simulink model "10_MCU_PMSM1_Trajectoire_dsPIC33CK_LVMC"  (R2023b)
settings: Solver=FixedStepDiscrete  StartTime=0.0  StopTime=10.0  FixedStep=5e-5  RelTol=1e-3  EnableMultiTasking=on
InitFcn:
  | %% Trajectoire Source
  | 
  | t0 = 0;
  | t1 = t0+0.1;
  | t2 = t1+0.1;
  | t3 = t2+0.5;
  | t4 = t3+0.2;
  | t5 = t4+0.5;
  | t6 = t5+0.2;
  | t7 = t6+0.1;
  | 
  | 
  | 
  | x = [t0 t1 t2 t3 t4 t5 t6 t7];
  | y = [0 0 0.25 0.25 1 1 0 0];
  | 
  | 
  | %% Trajectoire charge
  | t0 = 0;
  | t1 = t0+0.4;
  | t2 = t1+1e-2;
  | t3 = t2+0.1;
  | t4 = t3+1e-2;
  | t5 = 1.1;
  | t6 = t5+1e-2;
  | t7 = t6+0.1
  | t8 = t7+1e-2
  | t9 = 1.7;
  | x2 = [t0 t1 t2 t3 t4 t5 t6 t7 t8 t9];
  | y2 = [0 0 1 1 0 0 1 1 0 0];
undefined symbols (not defined in the file or in its folder): A0, A4, AN0, AN1, B0, B2, Bias1, Bias2, C12, C13, C14, C7, control, D11, D12, D13, D14, D5, D6, D7, diff, DiscIntNeverNeededParam, inverter, Max, MaxPer, model, ms, NumBits1, NumBits2, P20, P32, P55, P60, P61, P62, P69, P70, P71, P75, P76, P77, P78, Pin, pmsm, PosRange1, PosRange2, PWM1max, Resol, s, Slope1, Slope2, us
libraries: simulink x55, MCHP_Blockset x26
(part 4 of 4)

== system 10_MCU_PMSM1_Trajectoire_dsPIC33CK_LVMC/Park/Clarke ==
  note: Clark transform
      | $x_{\alpha\beta} = \frac{2}{3}\underbrace{\left[\begin{array}{ccc}1&-\frac{1}{2}&-\frac{1}{2}\\0&\frac{\sqrt{3}}{2}&-\frac{\sqrt{3}}{2}\end{array}\right]}_{C_{23}}x_{abc}$
      | if only 2 currents are measured since $x_a+x_b+x_c = 0$
      | $x_{abc} = \left[\begin{array}{cc}1 & 0\\0 & 1\\-1&-1\end{array}\right]x_{ab}$
      | leading to
      | $x_{\alpha\beta} = \underbrace{\left[\begin{array}{cc}1&0\\\frac{1}{\sqrt{3}}&\frac{2}{\sqrt{3}}\end{array}\right]}_{C_{22}}x_{ab}$
  xab(c) : Inport
  C1 : Gain  Gain=[1/sqrt(3) 2/sqrt(3)]  Multiplication=Matrix(K*u)  OutDataTypeStr=Inherit: Same as input
  Mux : Mux  Inputs=2
  Selector : Selector  InputPortWidth=2  IndexOptions=Index vector (dialog)  Indices=[1]  OutputSizes=1
  xalphabeta : Outport  VectorParamsAs1DForOutWhenUnconnected=off
  wires:
  C1/1 -> Mux/2
  Selector/1 -> Mux/1
  Mux/1 -> xalphabeta/1
  xab(c)/1 -> C1/1, Selector/1

== system 10_MCU_PMSM1_Trajectoire_dsPIC33CK_LVMC/Park/Park ==
  note: Park
      | $x_{dq} = P(\theta)^{-1}x_{\alpha\beta}\\ P(p\theta)^{-1} = \left[\begin{array}{cc}\cos(p\theta) & \sin(p\theta)\\ -\sin(p\theta) & \cos(p\theta) \end{array}\right]$
  xalphabeta : Inport  PortDimensions=2
  P(pth) : Inport  Port=2
  Data Type Duplicate2 : DataTypeDuplicate
  Park : Product  Multiplication=Matrix(*)  OutDataTypeStr=Inherit: Inherit via back propagation  RndMeth=Round
  xdq : Outport  VectorParamsAs1DForOutWhenUnconnected=off
  wires:
  P(pth)/1 -> Park/1
  xalphabeta/1 -> Park/2, Data Type Duplicate2/2
  Park/1 -> xdq/1, Data Type Duplicate2/1

== system 10_MCU_PMSM1_Trajectoire_dsPIC33CK_LVMC/Park inverse/Clarke Inverse ==
  note: Clarke inverse
  xalphabeta : Inport
  C23' : Gain  Gain=|  Multiplication=Matrix(K*u)  OutDataTypeStr=Inherit: Inherit via back propagation  RndMeth=Round
      | [1   -1/2        -1/2;
      |         0   sqrt(3)/2   -sqrt(3)/2]'
  xabc : Outport  VectorParamsAs1DForOutWhenUnconnected=off
  wires:
  xalphabeta/1 -> C23'/1
  C23'/1 -> xabc/1

== system 10_MCU_PMSM1_Trajectoire_dsPIC33CK_LVMC/Park inverse/Park inverse ==
  note: Inverse Park
      | $x_{\alpha\beta} = P(p\theta)x_{dq}\\ P(p\theta) = \left[\begin{array}{cc}\cos(p\theta) & -\sin(p\theta)\\ \sin(p\theta) & \cos(p\theta) \end{array}\right]$
  xdq : Inport
  P(pth) : Inport  Port=2
  Data Type Duplicate2 : DataTypeDuplicate
  Transpose : Math  Operator=transpose
  Transpose1 : Math  Operator=transpose
  xalpha sin(pth)1 : Product  Multiplication=Matrix(*)  OutDataTypeStr=Inherit: Inherit via back propagation  RndMeth=Round
  xalpahbeta : Outport  VectorParamsAs1DForOutWhenUnconnected=off
  wires:
  P(pth)/1 -> xalpha sin(pth)1/2
  Transpose1/1 -> xalpahbeta/1
  Transpose/1 -> Data Type Duplicate2/2, xalpha sin(pth)1/1
  xdq/1 -> Transpose/1
  xalpha sin(pth)1/1 -> Data Type Duplicate2/1, Transpose1/1

== system 10_MCU_PMSM1_Trajectoire_dsPIC33CK_LVMC/Selector/Direction Toggle ==
  in : Inport
  Change when button is pressed : simulink/Logic and Bit Operations/Detect Decrease  vinit=0.0  OutDataTypeStr=uint8
  Logical Operator : Logic  Operator=XOR  AllPortsSameDT=off  OutDataTypeStr=boolean
  Unit Delay : UnitDelay  SampleTime=-1  HasFrameUpgradeWarning=on
  Toggle : Outport  VectorParamsAs1DForOutWhenUnconnected=off
  wires:
  Logical Operator/1 -> Unit Delay/1, Toggle/1  "Toggle"
  in/1 -> Change when button is pressed/1
  Change when button is pressed/1 -> Logical Operator/1
  Unit Delay/1 -> Logical Operator/2

== system 10_MCU_PMSM1_Trajectoire_dsPIC33CK_LVMC/Selector/Mode Toggle ==
  state : Inport
  Bitwise Operator : simulink/Logic and Bit Operations/Bitwise Operator  logicop=AND  UseBitMask=on  BitMask=1  BitMaskRealWorld=Stored Integer
  Change when button is pressed : simulink/Logic and Bit Operations/Detect Decrease  vinit=0.0  OutDataTypeStr=uint8
  Sum : Sum  OutDataTypeStr=uint16  AccumDataTypeStr=uint16
  Unit Delay : UnitDelay  SampleTime=-1  HasFrameUpgradeWarning=on
  Mode : Outport  PortDimensions=1  VectorParamsAs1DForOutWhenUnconnected=off
  wires:
  Change when button is pressed/1 -> Sum/1
  Bitwise Operator/1 -> Mode/1, Unit Delay/1
  Unit Delay/1 -> Sum/2
  Sum/1 -> Bitwise Operator/1
  state/1 -> Change when button is pressed/1

== system 10_MCU_PMSM1_Trajectoire_dsPIC33CK_LVMC/Selector/On//Off Toggle ==
  in : Inport
  Change when button is pressed : simulink/Logic and Bit Operations/Detect Decrease  vinit=0.0  OutDataTypeStr=uint8
  Logical Operator : Logic  Operator=XOR  AllPortsSameDT=off  OutDataTypeStr=boolean
  Unit Delay : UnitDelay  SampleTime=-1  HasFrameUpgradeWarning=on
  Toggle : Outport  VectorParamsAs1DForOutWhenUnconnected=off
  wires:
  Unit Delay/1 -> Logical Operator/2
  Change when button is pressed/1 -> Logical Operator/1
  in/1 -> Change when button is pressed/1
  Logical Operator/1 -> Unit Delay/1, Toggle/1  "Toggle"

== system 10_MCU_PMSM1_Trajectoire_dsPIC33CK_LVMC/Selector/Subsystem1 ==
  Enable : EnablePort  StatesWhenEnabling=reset
  1-D Lookup Table : Lookup_n-D  NumberOfTableDimensions=1  BreakpointsForDimension1=x  Table=y  ExtrapMethod=Clip  InternalRulePriority=Speed  OutDataTypeStr=fixdt(1,16,14)  RndMeth=Simplest
  Constant : Constant  OutDataTypeStr=int16  SampleTime=0.001
  Discrete-Time Integrator : DiscreteIntegrator  SampleTime=0.001  OutDataTypeStr=fixdt(1,32,20)  SaturateOnIntegerOverflow=on  LimitOutput=on  UpperSaturationLimit=100  LowerSaturationLimit=0  ICPrevOutput=DiscIntNeverNeededParam  ICPrevScaledInput=DiscIntNeverNeededParam
  Gain : Gain  Gain=1.7/10  OutMax=[100]  OutDataTypeStr=fixdt(1,16,7)
  Mode1 : Outport
  wires:
  Discrete-Time Integrator/1 -> Gain/1
  Gain/1 -> 1-D Lookup Table/1
  1-D Lookup Table/1 -> Mode1/1
  Constant/1 -> Discrete-Time Integrator/1

== system 10_MCU_PMSM1_Trajectoire_dsPIC33CK_LVMC/Selector/Subsystem2 ==
  In1 : Inport
  Trigger : TriggerPort  VariantControl=(inherit)  PortDimensions=1
  UART Tx : MCHP_Blockset/BUS UART/UART Tx  UART_REF=1  ORDERING=None  AllOrNothing=off  SampleTime=-1  MCHP_MASTERLINK=MCU_logTrajectoire_dsPIC33CK_LVMC/BOARD dsPIC33CK LVMC/Microchip Master  NSend_Input=off  UART_String=off  NSend_Output=off
      settings: SourceProductName=MPLAB Device Blocks for Simulink
  wires:
  In1/1 -> UART Tx/1

== system 10_MCU_PMSM1_Trajectoire_dsPIC33CK_LVMC/Selector/Subsystem3 ==
  In1 : Inport
  Trigger : TriggerPort  TriggerType=falling  VariantControl=(inherit)  PortDimensions=1
  UART Tx : MCHP_Blockset/BUS UART/UART Tx  UART_REF=1  ORDERING=None  AllOrNothing=off  SampleTime=-1  MCHP_MASTERLINK=MCU_logTrajectoire_dsPIC33CK_LVMC/BOARD dsPIC33CK LVMC/Microchip Master  NSend_Input=off  UART_String=off  NSend_Output=off
      settings: SourceProductName=MPLAB Device Blocks for Simulink
  wires:
  In1/1 -> UART Tx/1

== system 10_MCU_PMSM1_Trajectoire_dsPIC33CK_LVMC/BOARD dsPIC33CK LVMC/Center & sign reversal/Downsample Averaged 2000 samples remove bias ==
  note: DownSample & Average by changing data scaling
  In1 : Inport
  Enable : EnablePort
  Compare To Constant : simulink/Logic and Bit Operations/Compare To Constant  relop===  const=1  OutDataTypeStr=boolean
  Counter Limited : simulink/Sources/Counter Limited  uplimit=DownSample-1  tsamp=-1
  Data Type Duplicate : DataTypeDuplicate
  Data Type Propagation : simulink/Signal Attributes/Data Type Propagation  PropDataType=fixdt(1, 16)  IfRefDouble=double  IfRefSingle=single  IsSigned=IsSigned1 or IsSigned2  NumBitsBase=NumBits1+NumBits2  NumBitsMult=1  NumBitsAdd=0  NumBitsAllowFinal=1:128  PropScaling=2^-10  ValuesUsedBestPrec=[5 -7]  SlopeBase=Slope1  SlopeMult=1  SlopeAdd=0  BiasBase=Bias1  BiasMult=1  BiasAdd=0
  Data Type Propagation1 : simulink/Signal Attributes/Data Type Propagation  PropDataType=fixdt(1, 16)  IfRefDouble=double  IfRefSingle=single  IsSigned=IsSigned1 or IsSigned2  NumBitsBase=NumBits1+NumBits2  NumBitsMult=1  NumBitsAdd=0  NumBitsAllowFinal=1:128  PropScaling=2^-10  ValuesUsedBestPrec=[5 -7]  SlopeBase=PosRange1  SlopeMult=1  SlopeAdd=0  BiasBase=Bias1  BiasMult=1  BiasAdd=0
  Discrete-Time Integrator : DiscreteIntegrator  IntegratorMethod=Accumulation: Backward Euler  gainval=1  ExternalReset=sampled level  SampleTime=-1  OutDataTypeStr=Inherit: Inherit via back propagation  ICPrevOutput=DiscIntNeverNeededParam  ICPrevScaledInput=DiscIntNeverNeededParam
  Gain : Gain  Gain=1/DownSample  OutDataTypeStr=Inherit: Inherit via back propagation  RndMeth=Round
  Gain1 : Gain  Gain=1/DownSample  OutDataTypeStr=Inherit: Inherit via back propagation
  Rate Transition1 : RateTransition  OutPortSampleTimeOpt=Multiple of input port sample time  OutPortSampleTimeMultiple=DownSample  OutPortSampleTime=DownSample
  Rate Transition3 : RateTransition  OutPortSampleTimeOpt=Multiple of input port sample time  OutPortSampleTimeMultiple=DownSample  OutPortSampleTime=DownSample
  Terminator : Terminator
  Out1 : Outport  VectorParamsAs1DForOutWhenUnconnected=off
  wires:
  Gain1/1 -> Data Type Propagation1/3, Terminator/1
  Rate Transition1/1 -> Data Type Duplicate/1, Data Type Propagation1/1, Data Type Propagation1/2
  Gain/1 -> Out1/1, Data Type Duplicate/2
  Counter Limited/1 -> Compare To Constant/1
  Discrete-Time Integrator/1 -> Rate Transition3/1, Data Type Propagation/3
  Compare To Constant/1 -> Discrete-Time Integrator/2
  In1/1 -> Data Type Propagation/1, Data Type Propagation/2, Discrete-Time Integrator/1, Rate Transition1/1
  Rate Transition3/1 -> Gain/1, Gain1/1

== system 10_MCU_PMSM1_Trajectoire_dsPIC33CK_LVMC/BOARD dsPIC33CK LVMC/Timing Analysis/Downsample Averaged2 ==
  note: DownSample & Average by changing data scaling
  In1 : Inport
  Compare To Constant : simulink/Logic and Bit Operations/Compare To Constant  relop===  const=1  OutDataTypeStr=boolean
  Counter Limited : simulink/Sources/Counter Limited  uplimit=DownSample-1  tsamp=-1
  Data Type Duplicate : DataTypeDuplicate
  Data Type Propagation : simulink/Signal Attributes/Data Type Propagation  PropDataType=fixdt(1, 16)  IfRefDouble=double  IfRefSingle=single  IsSigned=IsSigned1 or IsSigned2  NumBitsBase=NumBits1+NumBits2  NumBitsMult=1  NumBitsAdd=0  NumBitsAllowFinal=1:128  PropScaling=2^-10  ValuesUsedBestPrec=[5 -7]  SlopeBase=Slope1  SlopeMult=1  SlopeAdd=0  BiasBase=Bias1  BiasMult=1  BiasAdd=0
  Data Type Propagation1 : simulink/Signal Attributes/Data Type Propagation  PropDataType=fixdt(1, 16)  IfRefDouble=double  IfRefSingle=single  IsSigned=IsSigned1 or IsSigned2  NumBitsBase=NumBits1+NumBits2  NumBitsMult=1  NumBitsAdd=0  NumBitsAllowFinal=1:128  PropScaling=2^-10  ValuesUsedBestPrec=[5 -7]  SlopeBase=PosRange1  SlopeMult=1  SlopeAdd=0  BiasBase=Bias1  BiasMult=1  BiasAdd=0
  Discrete-Time Integrator : DiscreteIntegrator  IntegratorMethod=Accumulation: Backward Euler  gainval=1  ExternalReset=sampled level  SampleTime=-1  OutDataTypeStr=Inherit: Inherit via back propagation  ICPrevOutput=DiscIntNeverNeededParam  ICPrevScaledInput=DiscIntNeverNeededParam
  Gain : Gain  Gain=1/DownSample  OutDataTypeStr=Inherit: Inherit via back propagation
  Gain1 : Gain  Gain=1/DownSample  OutDataTypeStr=Inherit: Inherit via back propagation
  Rate Transition1 : RateTransition  Deterministic=off  OutPortSampleTime=[InputSampleTime * DownSample]
  Rate Transition3 : RateTransition  OutPortSampleTime=[InputSampleTime * DownSample]
  Terminator : Terminator
  Out1 : Outport  VectorParamsAs1DForOutWhenUnconnected=off
  wires:
  Rate Transition3/1 -> Gain1/1, Gain/1
  In1/1 -> Discrete-Time Integrator/1, Rate Transition1/1, Data Type Propagation/2, Data Type Propagation/1
  Compare To Constant/1 -> Discrete-Time Integrator/2
  Discrete-Time Integrator/1 -> Data Type Propagation/3, Rate Transition3/1
  Counter Limited/1 -> Compare To Constant/1
  Gain/1 -> Data Type Duplicate/2, Out1/1
  Rate Transition1/1 -> Data Type Propagation1/2, Data Type Propagation1/1, Data Type Duplicate/1
  Gain1/1 -> Data Type Propagation1/3, Terminator/1

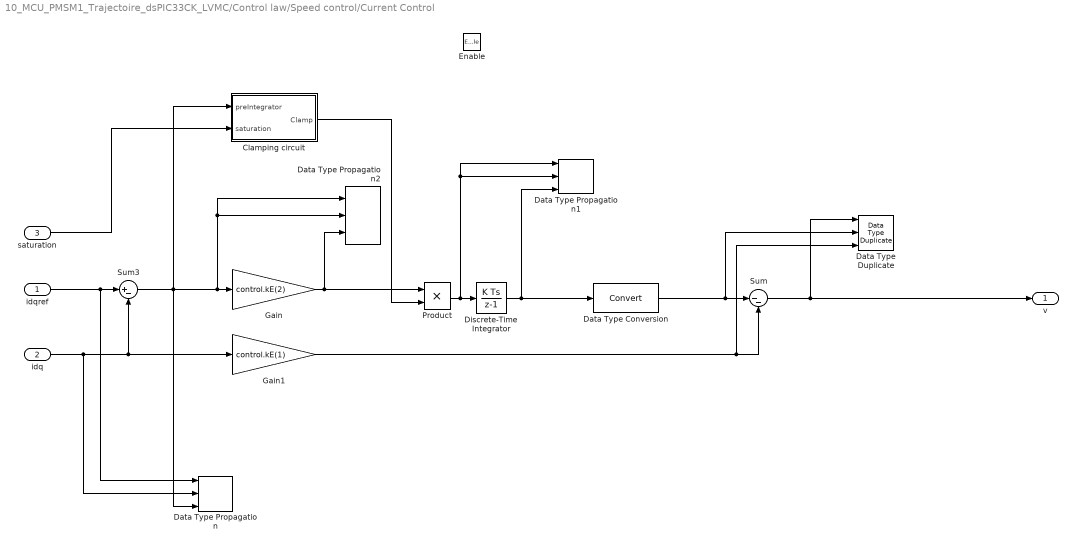
== system 10_MCU_PMSM1_Trajectoire_dsPIC33CK_LVMC/Control law/Speed control/Current Control ==
  idqref : Inport
  idq : Inport  Port=2
  saturation : Inport  Port=3
  Enable : EnablePort  StatesWhenEnabling=reset
  Clamping circuit : Subsystem
  Data Type Duplicate : DataTypeDuplicate  NumInputPorts=3
  Data Type Propagation : simulink/Signal Attributes/Data Type Propagation  PropDataType=fixdt(1, 16)  IfRefDouble=double  IfRefSingle=single  IsSigned=IsSigned1 or IsSigned2  NumBitsBase=max([NumBits1 NumBits2])  NumBitsMult=1  NumBitsAdd=0  NumBitsAllowFinal=1:128  PropScaling=2^-(15-ceil(log2(2*inverter.iMax)))  ValuesUsedBestPrec=[5 -7]  SlopeBase=max([PosRange1 PosRange2])  SlopeMult=2  SlopeAdd=0  BiasBase=Bias1  BiasMult=1  BiasAdd=0
  Data Type Propagation1 : simulink/Signal Attributes/Data Type Propagation  PropDataType=fixdt(1, 16)  IfRefDouble=single  IfRefSingle=single  IsSigned=IsSigned1 or IsSigned2  NumBitsBase=NumBits1+NumBits2  NumBitsMult=1  NumBitsAdd=0  NumBitsAllowFinal=1:128  PropScalingMode=Specify via dialog  PropScaling=2^-23  ValuesUsedBestPrec=[5 -7]  SlopeBase=min([Slope1 Slope2])  SlopeMult=1  SlopeAdd=0  BiasBase=Bias1  BiasMult=1  BiasAdd=0
  Data Type Propagation2 : simulink/Signal Attributes/Data Type Propagation  PropDataType=fixdt(1, 16)  IfRefDouble=double  IfRefSingle=single  IsSigned=TRUE  NumBitsBase=max([NumBits1 NumBits2])  NumBitsMult=1  NumBitsAdd=0  NumBitsAllowFinal=[1:128]  PropScaling=2^-(15-ceil(log2(inverter.vDC/sqrt(3))))  ValuesUsedBestPrec=[100 -100]  SlopeBase=max([PosRange1 PosRange2])  SlopeMult=abs(control.kE(2))  SlopeAdd=0  BiasBase=Bias1  BiasMult=1  BiasAdd=0
  Data Type Conversion : DataTypeConversion  SaturateOnIntegerOverflow=off  RndMeth=Floor
  Discrete-Time Integrator : DiscreteIntegrator  SampleTime=-1  OutDataTypeStr=Inherit: Inherit via back propagation  SaturateOnIntegerOverflow=on  ICPrevOutput=DiscIntNeverNeededParam  ICPrevScaledInput=DiscIntNeverNeededParam
  Gain : Gain  Gain=control.kE(2)  OutDataTypeStr=Inherit: Inherit via back propagation  SaturateOnIntegerOverflow=on
  Gain1 : Gain  Gain=control.kE(1)  OutDataTypeStr=Inherit: Inherit via back propagation  SaturateOnIntegerOverflow=on
  Product : Product  OutDataTypeStr=Inherit: Same as first input
  Sum : Sum  Inputs=|--  OutDataTypeStr=Inherit: Inherit via back propagation  SaturateOnIntegerOverflow=on
  Sum3 : Sum  Inputs=|+-  OutDataTypeStr=Inherit: Inherit via back propagation  SaturateOnIntegerOverflow=on
  v : Outport  VectorParamsAs1DForOutWhenUnconnected=off
  wires:
  Data Type Conversion/1 -> Sum/1, Data Type Duplicate/2
  Sum/1 -> v/1, Data Type Duplicate/1
  idqref/1 -> Sum3/1, Data Type Propagation/1
  idq/1 -> Sum3/2, Gain1/1, Data Type Propagation/2
  Discrete-Time Integrator/1 -> Data Type Conversion/1, Data Type Propagation1/3
  Gain1/1 -> Sum/2, Data Type Duplicate/3
  saturation/1 -> Clamping circuit/2(saturation)
  Product/1 -> Data Type Propagation1/2, Data Type Propagation1/1, Discrete-Time Integrator/1
  Clamping circuit/1(Clamp) -> Product/2
  Gain/1 -> Data Type Propagation2/3, Product/1
  Sum3/1 -> Gain/1, Data Type Propagation2/2, Data Type Propagation2/1, Data Type Propagation/3, Clamping circuit/1(preIntegrator)

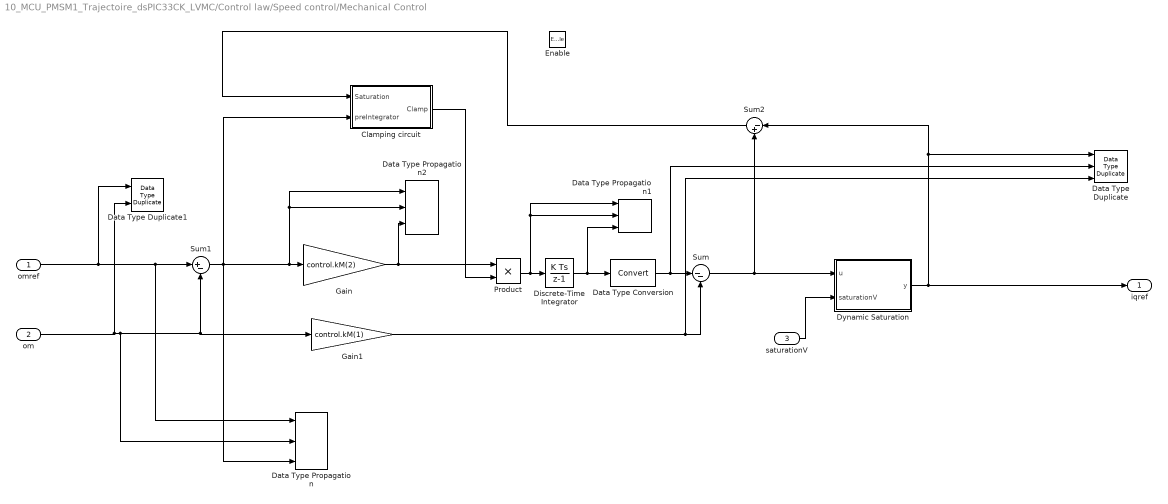
== system 10_MCU_PMSM1_Trajectoire_dsPIC33CK_LVMC/Control law/Speed control/Mechanical Control ==
  omref : Inport
  om : Inport  Port=2
  saturationV : Inport  Port=3
  Enable : EnablePort  StatesWhenEnabling=reset
  Clamping circuit : Subsystem
  Data Type Duplicate : DataTypeDuplicate  NumInputPorts=3
  Data Type Duplicate1 : DataTypeDuplicate
  Data Type Propagation : simulink/Signal Attributes/Data Type Propagation  PropDataType=fixdt(1, 16)  IfRefDouble=double  IfRefSingle=single  IsSigned=IsSigned1 or IsSigned2  NumBitsBase=max([NumBits1 NumBits2])  NumBitsMult=1  NumBitsAdd=0  NumBitsAllowFinal=1:128  PropScaling=2^-(15-ceil(log2(2*pmsm.omegaMax)))  ValuesUsedBestPrec=[5 -7]  SlopeBase=max([PosRange1 PosRange2])  SlopeMult=2  SlopeAdd=0  BiasBase=Bias1  BiasMult=1  BiasAdd=0
  Data Type Propagation1 : simulink/Signal Attributes/Data Type Propagation  PropDataType=fixdt(1, 16)  IfRefDouble=single  IfRefSingle=single  IsSigned=IsSigned1 or IsSigned2  NumBitsBase=NumBits1+NumBits2  NumBitsMult=1  NumBitsAdd=0  NumBitsAllowFinal=1:128  PropScalingMode=Specify via dialog  PropScaling=2^-23  ValuesUsedBestPrec=[5 -7]  SlopeBase=min([Slope1 Slope2])  SlopeMult=1  SlopeAdd=0  BiasBase=Bias1  BiasMult=1  BiasAdd=0
  Data Type Propagation2 : simulink/Signal Attributes/Data Type Propagation  PropDataType=fixdt(1, 16)  IfRefDouble=double  IfRefSingle=single  IsSigned=TRUE  NumBitsBase=max([NumBits1 NumBits2])  NumBitsMult=1  NumBitsAdd=0  NumBitsAllowFinal=[1:128]  PropScaling=2^-(15-ceil(log2(inverter.vDC/sqrt(3))))  ValuesUsedBestPrec=[100 -100]  SlopeBase=max([PosRange1 PosRange2])  SlopeMult=abs(control.kM(2))  SlopeAdd=0  BiasBase=Bias1  BiasMult=1  BiasAdd=0
  Data Type Conversion : DataTypeConversion  SaturateOnIntegerOverflow=off  RndMeth=Floor
  Discrete-Time Integrator : DiscreteIntegrator  SampleTime=-1  OutDataTypeStr=Inherit: Inherit via back propagation  SaturateOnIntegerOverflow=on  ICPrevOutput=DiscIntNeverNeededParam  ICPrevScaledInput=DiscIntNeverNeededParam
  Dynamic Saturation : Subsystem
  Gain : Gain  Gain=control.kM(2)  OutDataTypeStr=Inherit: Inherit via back propagation  SaturateOnIntegerOverflow=on
  Gain1 : Gain  Gain=control.kM(1)  OutDataTypeStr=Inherit: Inherit via back propagation  SaturateOnIntegerOverflow=on
  Product : Product  OutDataTypeStr=Inherit: Same as first input
  Sum : Sum  Inputs=|--  OutDataTypeStr=Inherit: Inherit via back propagation  SaturateOnIntegerOverflow=on
  Sum1 : Sum  Inputs=|+-  OutDataTypeStr=Inherit: Inherit via back propagation
  Sum2 : Sum  Inputs=|-+  SaturateOnIntegerOverflow=on  OutDataTypeStr=Inherit: Same as first input
  iqref : Outport  VectorParamsAs1DForOutWhenUnconnected=off
  wires:
  Data Type Conversion/1 -> Sum/1, Data Type Duplicate/2
  Dynamic Saturation/1(y) -> Sum2/1, Data Type Duplicate/1, iqref/1
  Sum/1 -> Sum2/2, Dynamic Saturation/1(u)
  Discrete-Time Integrator/1 -> Data Type Conversion/1, Data Type Propagation1/3
  om/1 -> Data Type Duplicate1/2, Sum1/2, Gain1/1, Data Type Propagation/2
  omref/1 -> Sum1/1, Data Type Propagation/1, Data Type Duplicate1/1
  Clamping circuit/1(Clamp) -> Product/2
  Sum2/1 -> Clamping circuit/1(Saturation)
  Gain1/1 -> Sum/2, Data Type Duplicate/3
  saturationV/1 -> Dynamic Saturation/2(saturationV)
  Product/1 -> Data Type Propagation1/2, Data Type Propagation1/1, Discrete-Time Integrator/1
  Gain/1 -> Data Type Propagation2/3, Product/1
  Sum1/1 -> Data Type Propagation2/1, Data Type Propagation2/2, Gain/1, Clamping circuit/2(preIntegrator), Data Type Propagation/3

== system 10_MCU_PMSM1_Trajectoire_dsPIC33CK_LVMC/Control law/Voltage Saturation2/1//sqrt(u) ==
  u : Inport
  Calc 1/sqrt(u) : Subsystem
  Compare To Constant : simulink/Logic and Bit Operations/Compare To Constant  relop===  const=1  OutDataTypeStr=boolean
  Compare To Constant1 : simulink/Logic and Bit Operations/Compare To Constant  relop===  const=0  OutDataTypeStr=boolean
  "LUT 1/sqrt(u) " : Subsystem
  Switch : Switch  Criteria=u2 > Threshold  SaturateOnIntegerOverflow=off  InputSameDT=off
  isSingle : Subsystem
  y : Outport
  wires:
  Compare To Constant/1 -> Calc 1/sqrt(u)/Enable
  Compare To Constant1/1 -> "LUT 1/sqrt(u) "/Enable
  Switch/1 -> y/1
  "LUT 1/sqrt(u) "/1(vdqsat1) -> Switch/3
  Calc 1/sqrt(u)/1(Out1) -> Switch/1
  isSingle/1(y) -> Switch/2, Compare To Constant/1, Compare To Constant1/1
  u/1 -> "LUT 1/sqrt(u) "/1(y), isSingle/1(u), Calc 1/sqrt(u)/1(u)

== system 10_MCU_PMSM1_Trajectoire_dsPIC33CK_LVMC/Control law/Voltage Saturation2/Norm L2 ==
  In1 : Inport
  Data Type Propagation : simulink/Signal Attributes/Data Type Propagation  PropDataType=fixdt(1, 16)  IfRefDouble=double  IfRefSingle=single  IsSigned=IsSigned1 or IsSigned2  NumBitsBase=max([NumBits1 NumBits2])  NumBitsMult=1  NumBitsAdd=0  NumBitsAllowFinal=1:128  PropScalingMode=Specify via dialog  PropScaling=2^-model.FracLen.volt2  ValuesUsedBestPrec=[5 -7]  SlopeBase=PosRange1*PosRange2  SlopeMult=1  SlopeAdd=0  BiasBase=max([Bias1 Bias2])  BiasMult=1  BiasAdd=0
  Dot Product : DotProduct  OutDataTypeStr=Inherit: Inherit via back propagation  SaturateOnIntegerOverflow=on
  y : Outport
  wires:
  In1/1 -> Data Type Propagation/1, Data Type Propagation/2, Dot Product/2, Dot Product/1
  Dot Product/1 -> Data Type Propagation/3, y/1

== system 10_MCU_PMSM1_Trajectoire_dsPIC33CK_LVMC/Control law/Voltage Saturation2/Square ==
  In1 : Inport
  Data Type Propagation : simulink/Signal Attributes/Data Type Propagation  PropDataType=fixdt(1, 16)  IfRefDouble=double  IfRefSingle=single  IsSigned=IsSigned1 or IsSigned2  NumBitsBase=max([NumBits1 NumBits2])  NumBitsMult=1  NumBitsAdd=0  NumBitsAllowFinal=1:128  PropScalingMode=Specify via dialog  PropScaling=2^-model.FracLen.volt2  ValuesUsedBestPrec=[5 -7]  SlopeBase=PosRange1*PosRange2  SlopeMult=1  SlopeAdd=0  BiasBase=max([Bias1 Bias2])  BiasMult=1  BiasAdd=0
  Square : Math  Operator=square  OutDataTypeStr=Inherit: Inherit via back propagation
  y : Outport
  wires:
  Square/1 -> Data Type Propagation/3, y/1
  In1/1 -> Square/1, Data Type Propagation/2, Data Type Propagation/1

== system 10_MCU_PMSM1_Trajectoire_dsPIC33CK_LVMC/Control law/Speed control/Current Control/Clamping circuit ==
  note: The clamping enable or disable the integral action.
  preIntegrator : Inport  DisableCoverage=on
  saturation : Inport  DisableCoverage=on  Port=2
  AND : Logic  Operator=OR  IconShape=distinctive  AllPortsSameDT=off  OutDataTypeStr=boolean
  Compare To Zero1 : simulink/Logic and Bit Operations/Compare To Zero  relop=<=  OutDataTypeStr=boolean
  Delay : Delay  DelayLength=1
  Demux : Demux  Outputs=2
  Multiply : Product
  Clamp : Outport  DisableCoverage=on  VectorParamsAs1DForOutWhenUnconnected=off
  wires:
  saturation/1 -> Delay/1
  Compare To Zero1/1 -> Demux/1
  Multiply/1 -> Compare To Zero1/1
  preIntegrator/1 -> Multiply/2
  AND/1 -> Clamp/1
  Demux/2 -> AND/2
  Demux/1 -> AND/1
  Delay/1 -> Multiply/1

== system 10_MCU_PMSM1_Trajectoire_dsPIC33CK_LVMC/Control law/Speed control/Mechanical Control/Clamping circuit ==
  note: The clamping enable or disable the integral action.
  Saturation : Inport  DisableCoverage=on
  preIntegrator : Inport  DisableCoverage=on  Port=2
  Compare To Zero1 : simulink/Logic and Bit Operations/Compare To Zero  relop=<=  OutDataTypeStr=boolean
  Delay : Delay  DelayLength=1  InitialCondition=0
  Multiply : Product
  Clamp : Outport  DisableCoverage=on  VectorParamsAs1DForOutWhenUnconnected=off
  wires:
  Delay/1 -> Multiply/1
  Saturation/1 -> Delay/1
  Multiply/1 -> Compare To Zero1/1
  preIntegrator/1 -> Multiply/2
  Compare To Zero1/1 -> Clamp/1

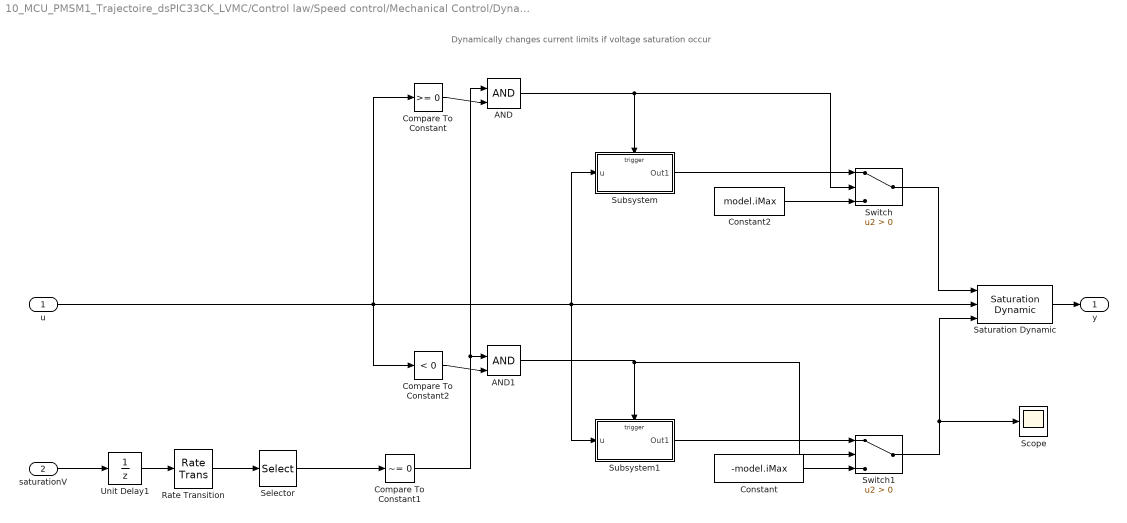
== system 10_MCU_PMSM1_Trajectoire_dsPIC33CK_LVMC/Control law/Speed control/Mechanical Control/Dynamic Saturation ==
  note: Dynamically changes current limits if voltage saturation occur
  u : Inport
  saturationV : Inport  Port=2
  AND : Logic  IconShape=distinctive  AllPortsSameDT=off  OutDataTypeStr=boolean
  AND1 : Logic  IconShape=distinctive  AllPortsSameDT=off  OutDataTypeStr=boolean
  Compare To Constant : simulink/Logic and Bit Operations/Compare To Constant  relop=>=  const=0  OutDataTypeStr=boolean
  Compare To Constant1 : simulink/Logic and Bit Operations/Compare To Constant  relop=~=  const=0  OutDataTypeStr=boolean
  Compare To Constant2 : simulink/Logic and Bit Operations/Compare To Constant  relop=<  const=0  OutDataTypeStr=boolean
  Constant : Constant  Value=-model.iMax  OutDataTypeStr=single  SampleTime=1e-3
  Constant2 : Constant  Value=model.iMax  OutDataTypeStr=single  SampleTime=1e-3
  Rate Transition : RateTransition  OutPortSampleTime=control.tsMeca
  Saturation Dynamic : simulink/Discontinuities/Saturation Dynamic  OutMin=[]  OutMax=[]  OutDataTypeStr=Inherit: Same as second input  OutDataType=fixdt(1, 16)  OutScaling=2^-10  DoSatur=off
  Scope : Scope
  Selector : Selector  InputPortWidth=2  IndexOptions=Index vector (dialog)  Indices=2  OutputSizes=1
  Subsystem : Subsystem
  Subsystem1 : Subsystem
  Switch : Switch  Criteria=u2 > Threshold  SaturateOnIntegerOverflow=off  InputSameDT=off
  Switch1 : Switch  Criteria=u2 > Threshold  SaturateOnIntegerOverflow=off  InputSameDT=off
  Unit Delay1 : UnitDelay  SampleTime=-1  HasFrameUpgradeWarning=on
  y : Outport
  wires:
  Switch/1 -> Saturation Dynamic/1
  u/1 -> Compare To Constant/1, Compare To Constant2/1, Subsystem/1(u), Subsystem1/1(u), Saturation Dynamic/2
  Saturation Dynamic/1 -> y/1
  saturationV/1 -> Unit Delay1/1
  Compare To Constant1/1 -> AND/1, AND1/1
  AND/1 -> Switch/2, Subsystem/Trigger
  Constant2/1 -> Switch/3
  Subsystem/1(Out1) -> Switch/1
  Compare To Constant2/1 -> AND1/2
  AND1/1 -> Subsystem1/Trigger, Switch1/2
  Subsystem1/1(Out1) -> Switch1/1
  Switch1/1 -> Scope/1, Saturation Dynamic/3
  Constant/1 -> Switch1/3
  Rate Transition/1 -> Selector/1
  Unit Delay1/1 -> Rate Transition/1
  Compare To Constant/1 -> AND/2
  Selector/1 -> Compare To Constant1/1

== system 10_MCU_PMSM1_Trajectoire_dsPIC33CK_LVMC/Control law/Voltage Saturation2/1//sqrt(u)/Calc 1//sqrt(u) ==
  u : Inport
  Enable : EnablePort
  Reciprocal : Product  Inputs=/
  Sqrt : Sqrt
  Out1 : Outport
  wires:
  Reciprocal/1 -> Out1/1
  u/1 -> Sqrt/1
  Sqrt/1 -> Reciprocal/1

== system 10_MCU_PMSM1_Trajectoire_dsPIC33CK_LVMC/Control law/Voltage Saturation2/1//sqrt(u)/LUT 1//sqrt(u)  ==
  y : Inport
  Enable : EnablePort
  1-D Lookup Table : Lookup_n-D  NumberOfTableDimensions=1  BreakpointsSpecification=Even spacing  BreakpointsForDimension1=model.math.LUTintsqrtx  BreakpointsForDimension1FirstPoint=model.math.LUTintsqrtx(1)  BreakpointsForDimension1Spacing=mean(diff(model.math.LUTintsqrtx))  IndexSearchMethod=Evenly spaced points  Table=model.math.LUTintsqrty  ExtrapMethod=Clip  DiagnosticForOutOfRangeInput=Error  UseLastTableValue=on  InternalRulePriority=Speed  OutDataTypeStr=Inherit: Inherit via back propagation  RndMeth=Simplest  FractionDataTypeStr=fixdt(1,16,15)  LockScale=on
  Data Type Propagation : simulink/Signal Attributes/Data Type Propagation  PropDataType=fixdt(1, 16)  IfRefDouble=double  IfRefSingle=single  IsSigned=IsSigned1 or IsSigned2  NumBitsBase=max([NumBits1 NumBits2])  NumBitsMult=1  NumBitsAdd=0  NumBitsAllowFinal=1:128  PropScalingMode=Specify via dialog  PropScaling=2^-model.FracLen.invsqrtvolt  ValuesUsedBestPrec=[5 -7]  SlopeBase=PosRange1*PosRange2  SlopeMult=1  SlopeAdd=0  BiasBase=max([Bias1 Bias2])  BiasMult=1  BiasAdd=0
  vdqsat1 : Outport
  wires:
  1-D Lookup Table/1 -> Data Type Propagation/3, vdqsat1/1
  y/1 -> 1-D Lookup Table/1, Data Type Propagation/2, Data Type Propagation/1

== system 10_MCU_PMSM1_Trajectoire_dsPIC33CK_LVMC/Control law/Voltage Saturation2/1//sqrt(u)/isSingle ==
  u : Inport
  Compare To Constant : simulink/Logic and Bit Operations/Compare To Constant  relop=>=  const=500000  OutDataTypeStr=boolean
  Constant1 : Constant  OutDataTypeStr=Inherit: Inherit via back propagation
  Data Type Duplicate : DataTypeDuplicate
  Data Type Propagation : simulink/Signal Attributes/Data Type Propagation  PropDataType=fixdt(1, 16)  IfRefDouble=double  IfRefSingle=single  IsSigned=IsSigned1 or IsSigned2  NumBitsBase=max([NumBits1 NumBits2])  NumBitsMult=1  NumBitsAdd=0  NumBitsAllowFinal=1:128  PropScaling=2^-10  ValuesUsedBestPrec=[5 -7]  SlopeBase=max([PosRange1 PosRange2])  SlopeMult=100000  SlopeAdd=0  BiasBase=Bias1  BiasMult=1  BiasAdd=0
  Data Type Conversion : DataTypeConversion  SaturateOnIntegerOverflow=off  RndMeth=Floor
  Gain : Gain  Gain=1000000  SaturateOnIntegerOverflow=on  OutDataTypeStr=Inherit: Same as input
  y : Outport
  wires:
  u/1 -> Data Type Duplicate/1
  Constant1/1 -> Gain/1, Data Type Duplicate/2
  Gain/1 -> Data Type Conversion/1, Data Type Propagation/2, Data Type Propagation/1
  Data Type Conversion/1 -> Data Type Propagation/3, Compare To Constant/1
  Compare To Constant/1 -> y/1

== system 10_MCU_PMSM1_Trajectoire_dsPIC33CK_LVMC/Control law/Speed control/Mechanical Control/Dynamic Saturation/Subsystem ==
  u : Inport
  Trigger : TriggerPort  VariantControl=(inherit)  PortDimensions=1
  Out1 : Outport
  wires:
  u/1 -> Out1/1

== system 10_MCU_PMSM1_Trajectoire_dsPIC33CK_LVMC/Control law/Speed control/Mechanical Control/Dynamic Saturation/Subsystem1 ==
  u : Inport
  Trigger : TriggerPort  VariantControl=(inherit)  PortDimensions=1
  Out1 : Outport
  wires:
  u/1 -> Out1/1
